simulink model "otter_LQR_speed01"  (R2020b)
settings: Solver=VariableStepAuto  StartTime=0.0  StopTime=150  RelTol=1e-3
values from neighbouring files (symbols this model uses):
  CI = [5 0 -1.03 -7.27e-24 -10 0 0.101 0.123 0.144 -1.94e-25 0.184 0]'    [trim_linmod_model.m]    (also in x0_LQR_speed.mat = [1 -1.58361738432e-05 -0.00255013289966 9.56198848895e-07 -1)
  F2 = [115.068306158 103.833436356 0 0 0 0 0 0 0 0 224.95575831 188.556022676 ... (24 elements, 2x12)]    [gain_LQR_speed.mat]
libraries: simulink x1, mssSimulink x1
settings Model: Creator=maxim  LastModifiedBy=maxim

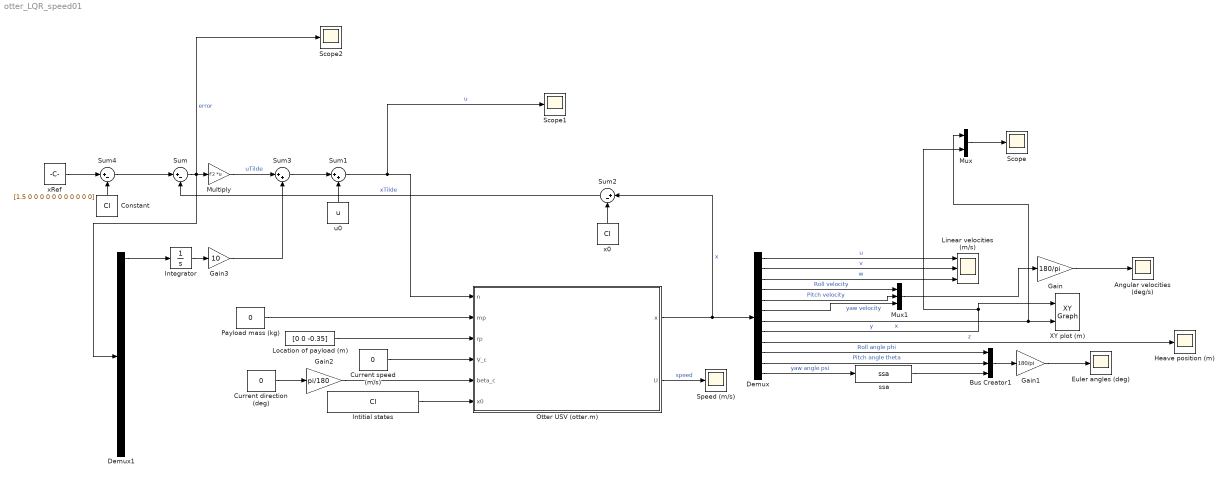
== system otter_LQR_speed01 ==
  Angular velocities (deg/s) : Scope
  Bus Creator1 : BusCreator  Inputs=3
  Constant : Constant  Value=CI
  Current direction (deg) : Constant  Value=0
  Current speed (m/s) : Constant  Value=0
  Demux : Demux  Outputs=12
  Demux1 : Demux  Outputs=12
  Euler angles (deg) : Scope
  Gain : Gain  Gain=180/pi
  Gain1 : Gain  Gain=180/pi
  Gain2 : Gain  Gain=pi/180
  Gain3 : Gain  Gain=10
  Heave position (m) : Scope
  Integrator : Integrator
  Intitial states : Constant  Value=CI
  Linear velocities (m/s) : Scope  NumInputPorts=3
  Location of payload (m) : Constant  Value=[0 0 -0.35]
  Multiply : Gain  Gain=F2  Multiplication=Matrix(K*u)
  Mux : Mux  Inputs=2
  Mux1 : Mux  Inputs=3
  "Otter USV (otter.m) " : Subsystem  AncestorBlock=mssSimulink/Marine craft models/Otter USV (otter.m)
      mask Display: image('otter.jpg'); % Use "Edit Image" on toolstrip to change.
  Payload mass (kg) : Constant  Value=0
  Scope : Scope
  Scope1 : Scope
  Scope2 : Scope
  Speed (m/s) : Scope
  Sum : Sum  Inputs=|+-
  Sum1 : Sum  Inputs=|++
  Sum2 : Sum  Inputs=|+-
  Sum3 : Sum  Inputs=|++
  Sum4 : Sum  Inputs=|+-
  XY plot (m) : simulink/Sinks/XY Graph  xmin=-200  xmax=200  ymin=-200  ymax=200  st=0.01
  "ssa   " : mssSimulink/Utilities/Math Operations/ssa  SystemSampleTime=-1  VariantActivationTime=update diagram  Latency=0  AutoFrameSizeCalculation=off
  u0 : Constant  Value=u
  x0 : Constant  Value=CI
  xRef : Constant  Value=[1.5 0 0 0 0 0 0 0 0 0 0 0]
  wires:
  Sum2/1 -> Sum/2  "xTilde"
  Demux/6 -> Mux1/3  "yaw velocity"
  Gain1/1 -> Euler angles (deg)/1
  Intitial states/1 -> "Otter USV (otter.m) "/6(x0)
  Sum/1 -> Demux1/1, Multiply/1, Scope2/1  "error"
  Demux/1 -> Linear velocities (m/s)/1  "u"
  Current speed (m/s)/1 -> "Otter USV (otter.m) "/4(V_c)
  u0/1 -> Sum1/2
  x0/1 -> Sum2/2
  Demux/5 -> Mux1/2  "Pitch velocity"
  Demux/7 -> Mux/1, XY plot (m)/2  "x"
  Demux/8 -> Mux/2, XY plot (m)/1  "y"
  Demux/4 -> Mux1/1  "Roll velocity"
  Gain/1 -> Angular velocities (deg/s)/1
  Gain2/1 -> "Otter USV (otter.m) "/5(beta_c)
  Demux/12 -> "ssa   "/1  "yaw angle psi"
  "ssa   "/1 -> Bus Creator1/3
  Mux1/1 -> Gain/1
  Current direction (deg)/1 -> Gain2/1
  Location of payload (m)/1 -> "Otter USV (otter.m) "/3(rp)
  Demux/9 -> Heave position (m)/1  "z"
  Demux/10 -> Bus Creator1/1  "Roll angle phi"
  Demux/2 -> Linear velocities (m/s)/2  "v"
  "Otter USV (otter.m) "/1(x) -> Sum2/1, Demux/1  "x"
  Demux/3 -> Linear velocities (m/s)/3  "w"
  "Otter USV (otter.m) "/2(U) -> Speed (m/s)/1  "speed"
  Payload mass (kg)/1 -> "Otter USV (otter.m) "/2(mp)
  Sum1/1 -> Scope1/1, "Otter USV (otter.m) "/1(n)  "u"
  Bus Creator1/1 -> Gain1/1
  Demux/11 -> Bus Creator1/2  "Pitch angle theta"
  Mux/1 -> Scope/1
  Demux1/1 -> Integrator/1
  Integrator/1 -> Gain3/1
  Multiply/1 -> Sum3/1  "uTilde"
  Gain3/1 -> Sum3/2
  Sum3/1 -> Sum1/1
  Sum4/1 -> Sum/1
  xRef/1 -> Sum4/1
  Constant/1 -> Sum4/2

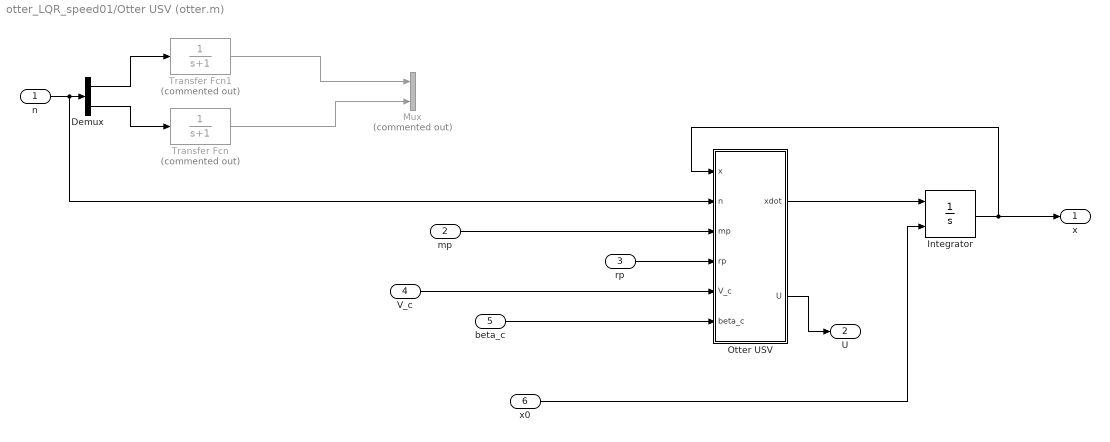
== system otter_LQR_speed01/Otter USV (otter.m)  ==
  n : Inport
  mp : Inport  Port=2
  rp : Inport  Port=3
  V_c : Inport  Port=4
  beta_c : Inport  Port=5
  x0 : Inport  Port=6
  Demux : Demux  Outputs=2
  Integrator : Integrator  InitialConditionSource=external  InitialCondition=[1 1]  UpperSaturationLimit=10  LowerSaturationLimit=-10  AbsoluteTolerance=1e-3
  Mux : Mux  Commented=on  Inputs=2
  Otter USV : MATLAB Function  TreatAsAtomicUnit=on
  Transfer Fcn : TransferFcn  Commented=on  Denominator=[1 1]
  Transfer Fcn1 : TransferFcn  Commented=on  Denominator=[1 1]
  x : Outport
  U : Outport  Port=2
  wires:
  Transfer Fcn1/1 -> Mux/1
  Transfer Fcn/1 -> Mux/2
  V_c/1 -> Otter USV/5(V_c)
  Otter USV/2(U) -> U/1
  mp/1 -> Otter USV/3(mp)
  Otter USV/1(xdot) -> Integrator/1
  Integrator/1 -> Otter USV/1(x), x/1
  beta_c/1 -> Otter USV/6(beta_c)
  rp/1 -> Otter USV/4(rp)
  x0/1 -> Integrator/2
  Demux/1 -> Transfer Fcn1/1
  Demux/2 -> Transfer Fcn/1
  n/1 -> Otter USV/2(n), Demux/1

== matlab function otter_LQR_speed01/Otter USV (otter.m) /Otter USV ==
  settings: updateMethod=DISCRETE
  data: x input; n input; xdot output; mp input; rp input; V_c input; beta_c input; U output
function [xdot, U] = fcn(x,n,mp,rp,V_c,beta_c)

[xdot,U] = otter(x,n,mp,rp,V_c,beta_c);

end
